simulink model "DC"  (R2021a)
settings: Solver=VariableStepAuto  StartTime=0.0  StopTime=10.0  RelTol=1e-3
values from neighbouring files (symbols this model uses):
  B = [27;-61.5;-21.5]    [gaussSir.m]    (also in motor.m = input('Enter value of B='); tf.m = [0;1])
  J = input('Enter value of J=')    [motor.m]
  Kb = input('Enter value of Kb=')    [motor.m]
  Kt = input('Enter value of Kt=')    [motor.m]
  L = input('L=')    [RLckt.m]    (also in motor.m = input('Enter value of L='))
  R = input('Enter value of R=')    [RC.m]    (also in RCckt.m = input('R='); RLckt.m = input('R='); motor.m)
settings Model: Creator=User  LastModifiedBy=User

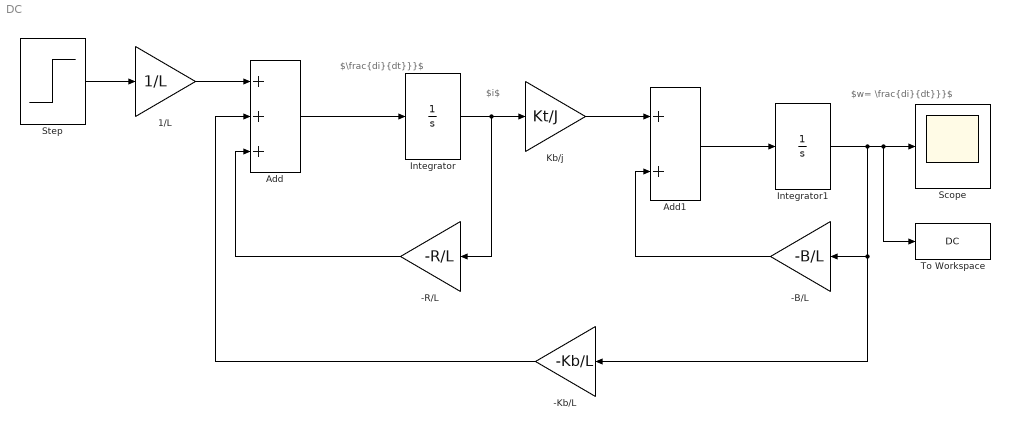
== system DC ==
  note: $\frac{di}{dt}}}$
  note: $w= \frac{di}{dt}}}$
  note: $i$
  -B/L : Gain  Gain=-B/L
  -Kb/L : Gain  Gain=-Kb/L
  -R/L : Gain  Gain=-R/L
  1/L : Gain  Gain=1/L
  Add : Sum  Inputs=+++
  Add1 : Sum
  Integrator : Integrator
  Integrator1 : Integrator
  Kb/j : Gain  Gain=Kt/J
  Scope : Scope
  Step : Step  SampleTime=0
  To Workspace : ToWorkspace  VariableName=DC  SaveFormat=Timeseries  SampleTime=-1
  wires:
  Add/1 -> Integrator/1
  Integrator/1 -> -R/L/1, Kb/j/1
  Kb/j/1 -> Add1/1
  Add1/1 -> Integrator1/1
  -B/L/1 -> Add1/2
  -R/L/1 -> Add/3
  -Kb/L/1 -> Add/2
  Integrator1/1 -> -Kb/L/1, -B/L/1, To Workspace/1, Scope/1
  1/L/1 -> Add/1
  Step/1 -> 1/L/1
